simulink model "simulation1"  (R2023b)
settings: Solver=VariableStepAuto  StartTime=0.0  StopTime=30  RelTol=1e-3
values from neighbouring files (symbols this model uses):
  b = x\y    [findM.m]    (also in simulation.m = 1/(G * K * H))
  G = 34.085968    [simulation.m]
  K = 0.3    [simulation.m]
  tau = (LDR * R) / (LDR + R) * C    [simulation.m]
  Ti = tau    [simulation.m]
settings Model: Creator=tomas  LastModifiedBy=tomas
settings DebuggingCC: AlgebraicLoopMsg=none

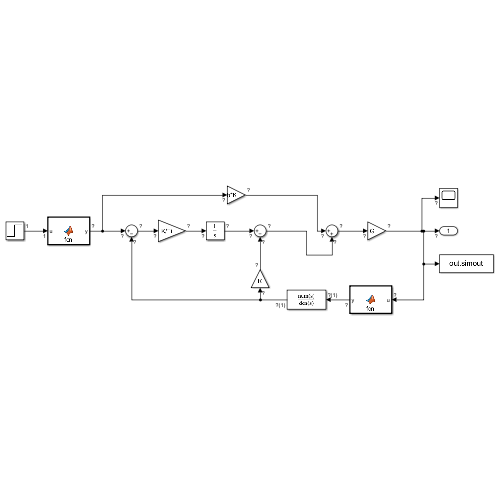
[thumbnail: Simulink's stored preview of the top-level diagram]
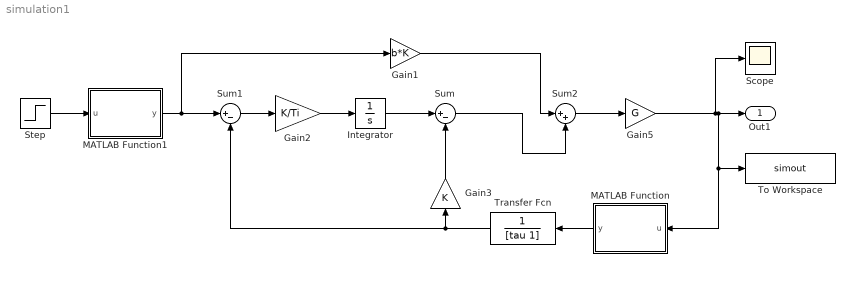
== system simulation1 ==
  Gain1 : Gain  Gain=b*K
  Gain2 : Gain  Gain=K/Ti
  Gain3 : Gain  Gain=K
  Gain5 : Gain  Gain=G
  Integrator : Integrator
  MATLAB Function : MATLAB Function  TreatAsAtomicUnit=on
  MATLAB Function1 : MATLAB Function  TreatAsAtomicUnit=on
  Scope : Scope
  Step : Step  Time=3  Before=0.3  After=20  SampleTime=0
  Sum : Sum  Inputs=|+-
  Sum1 : Sum  Inputs=|+-
  Sum2 : Sum  Inputs=|++
  To Workspace : ToWorkspace  VariableName=simout  SaveFormat=Timeseries  SampleTime=-1
  Transfer Fcn : TransferFcn  Denominator=[tau 1]
  Out1 : Outport
  wires:
  Step/1 -> MATLAB Function1/1(u)
  MATLAB Function1/1(y) -> Sum1/1, Gain1/1
  Gain2/1 -> Integrator/1
  Integrator/1 -> Sum/1
  Gain3/1 -> Sum/2
  Sum1/1 -> Gain2/1
  Gain5/1 -> MATLAB Function/1(u), To Workspace/1, Out1/1, Scope/1
  Gain1/1 -> Sum2/1
  Sum/1 -> Sum2/2
  Sum2/1 -> Gain5/1
  MATLAB Function/1(y) -> Transfer Fcn/1
  Transfer Fcn/1 -> Sum1/2, Gain3/1

== matlab function simulation1/MATLAB Function ==
  data: u input; y output
function y = fcn(u)
vcc = 3.3;
m = -0.9;
b = log10(225000) - m;
R = 10000;
LDR = power(10, (log10(complex(u)) * m + b));
vss =  vcc * R / (LDR + R);
H = vss/u;
y = H;

== matlab function simulation1/MATLAB Function1 ==
  data: u input; y output
function y = fcn(u)
vcc = 3.3;
m = -0.9;
b = log10(225000) - m;
R = 10000;
LDR = power(10, (log10(complex(u)) * m + b));
vss =  vcc * R / (LDR + R);
H = vss/u;
y = H;
